simulink model "m_seg_var_simulink"  (R2022a)
settings: Solver=FixedStepAuto  StartTime=0.0  StopTime=60  FixedStep=0.01  RelTol=1e-3
values from neighbouring files (symbols this model uses):
  A = importdata('matrix_A1lin.txt')    [m_seg_cte.m]    (also in m_seg_var.m)
  B2 = B    [m_seg_cte.m]    (also in m_seg_var.m = importdata('matrix_B1lin.txt'))
  C = importdata('matrix_C1.txt')    [m_seg_cte.m]    (also in m_seg_var.m)
  D = importdata('matrix_D1.txt')    [m_seg_cte.m]    (also in m_seg_var.m)
  K = place(A,B,p)    [m_seg_cte.m]    (also in m_seg_var.m = place(A,B2,p))
  Nu = N(7:9,:)    [m_seg_cte.m]
  Nx = N(1:6,:)    [m_seg_cte.m]
  xq_r = [q_r(2:4),x_r(4:6)]    [m_seg_var.m]
settings Model: Creator=gusta  LastModifiedBy=gusta

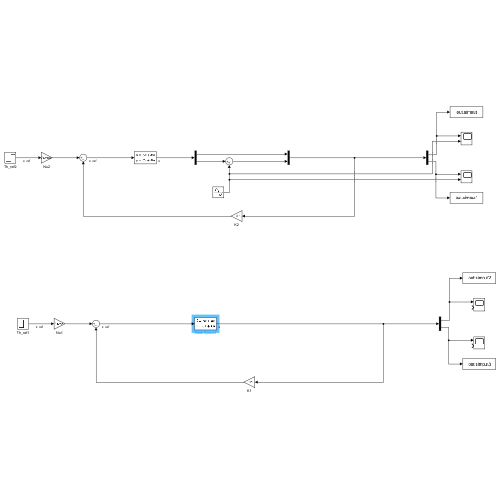
[thumbnail: Simulink's stored preview of the top-level diagram]
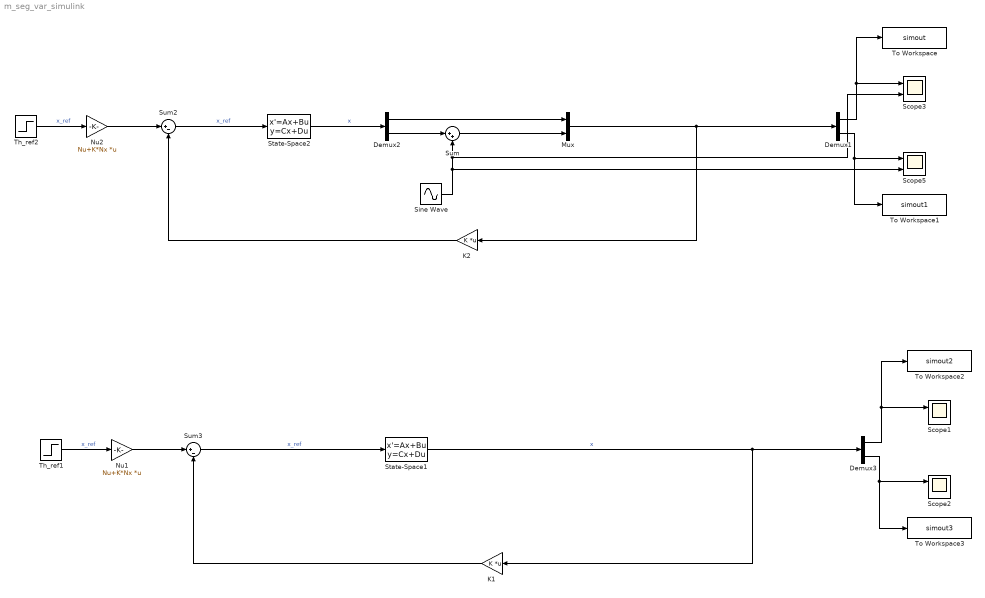
== system m_seg_var_simulink ==
  Demux1 : Demux  Outputs=2
  Demux2 : Demux  Outputs=2
  Demux3 : Demux  Outputs=2
  K1 : Gain  Gain=K  Multiplication=Matrix(K*u)
  K2 : Gain  Gain=K  Multiplication=Matrix(K*u)
  Mux : Mux  Inputs=2
  Nu1 : Gain  Gain=Nu+K*Nx  Multiplication=Matrix(K*u) (u vector)
  Nu2 : Gain  Gain=Nu+K*Nx  Multiplication=Matrix(K*u) (u vector)
  Scope{1..3,5} (4 alike) : Scope  NumInputPorts=2
  Sine Wave : Sin  Amplitude=0.02  Frequency=0.5  SampleTime=0
  State-Space1 : StateSpace  A=A  B=B2  C=C  D=D  InitialCondition=0
  State-Space2 : StateSpace  A=A  B=B2  C=C  D=D  InitialCondition=0
  Sum : Sum  Inputs=|++
  Sum2 : Sum  Inputs=|+-
  Sum3 : Sum  Inputs=|+-
  Th_ref1 : Step  Time=0  After=xq_r*0  SampleTime=0  VectorParams1D=off
  Th_ref2 : Step  Time=0  After=xq_r*0  SampleTime=0  VectorParams1D=off
  To Workspace : ToWorkspace  VariableName=simout  SaveFormat=Timeseries  SampleTime=-1
  To Workspace1 : ToWorkspace  VariableName=simout1  SaveFormat=Timeseries  SampleTime=-1
  To Workspace2 : ToWorkspace  VariableName=simout2  SaveFormat=Timeseries  SampleTime=-1
  To Workspace3 : ToWorkspace  VariableName=simout3  SaveFormat=Timeseries  SampleTime=-1
  wires:
  Demux1/2 -> To Workspace1/1, Scope5/1
  Demux1/1 -> To Workspace/1, Scope3/1
  K2/1 -> Sum2/2
  Th_ref2/1 -> Nu2/1  "x_ref"
  Nu2/1 -> Sum2/1
  Sum2/1 -> State-Space2/1  "x_ref"
  Sine Wave/1 -> Scope5/2, Scope3/2, Sum/2
  State-Space2/1 -> Demux2/1  "x"
  Mux/1 -> K2/1, Demux1/1
  Demux2/1 -> Mux/1
  Demux2/2 -> Sum/1
  Sum/1 -> Mux/2
  Demux3/1 -> To Workspace2/1, Scope1/1
  Th_ref1/1 -> Nu1/1  "x_ref"
  Demux3/2 -> To Workspace3/1, Scope2/1
  Sum3/1 -> State-Space1/1  "x_ref"
  Nu1/1 -> Sum3/1
  K1/1 -> Sum3/2
  State-Space1/1 -> K1/1, Demux3/1  "x"
